simulink model "gm_soc_dvbs2_fpga"  (R2025b)
settings: Solver=VariableStepAuto  StartTime=0.0  StopTime=10.0  RelTol=1e-3
InitFcn:
  | soc_dvbs2_init;
undefined symbols (not defined in the file or in its folder): Add, coefficientsLog, coefficientsSqrt1, coefficientsSqrt2, dataBits, Deinterleaver, designMultirateFIR, noisePow, Shift, Short, soc_dvbs2_designFIRFilter, soc_dvbs2_txPacketBits, syncWord, txDataOut, txFiltCoeff, XData
libraries: simulink x304, hdlsllib x265, dspsigops x15, dsphdlfiltering2 x8, hdlmdlgenlib x6, dsphdlsigops2 x5, commseqgen3 x5, dsphdlmathfun2 x3, hwlogicconnlib x2, whdledac x2, commhdlcrc x2, whdlutilities x1
(part 36 of 36)

== system gm_soc_dvbs2_fpga/DVBS2/DVBS2 TxRx/DVB-S2 HDL Receiver/Synchronizer and PL Header Decoder/Time Frequency and Coarse Phase Synchronizer/Fine Frequency Synchronizer/Modified L and R Algorithm/L and R Algorithm 18 point/Compute R(m) for 13 to 18/Compute R(m)_3/Complex Multiplier ==
  In1 : Inport  OutDataTypeStr=fixdt(1, 16, 11)  PortDimensions=1  SampleTime=2.5e-07
      settings: SignalType=complex
  In2 : Inport  Port=2  OutDataTypeStr=fixdt(1, 16, 11)  PortDimensions=1  SampleTime=2.5e-07
      settings: SignalType=complex
  AddADn : Sum  Inputs=++|  OutDataTypeStr=fixdt(1, 33, 22)
  AddAUp : Sum  Inputs=|+-  OutDataTypeStr=fixdt(1, 33, 22)
  AddBCtr : Sum  Inputs=+|+  OutDataTypeStr=fixdt(1, 17, 11)
  AddBDn : Sum  Inputs=|+-  OutDataTypeStr=fixdt(1, 17, 11)
  AddBUp : Sum  Inputs=++|  OutDataTypeStr=fixdt(1, 17, 11)
  Complex to Real-Imag : ComplexToRealImag
  Complex to Real-Imag1 : ComplexToRealImag
  Delay{1..5,8..20} (18 alike) : Delay  DelayLength=1
  Delay{6..7,21..27} (9 alike) : Delay
  Product : Product  OutDataTypeStr=fixdt(1, 33, 22)
  Product1 : Product  OutDataTypeStr=fixdt(1, 33, 22)
  Product2 : Product  OutDataTypeStr=fixdt(1, 33, 22)
  Real-Imag to Complex : RealImagToComplex
  Out1 : Outport  SampleTime=2.5e-07  VectorParamsAs1DForOutWhenUnconnected=off
  wires:
  Delay9/1 -> AddBUp/1
  Delay26/1 -> Delay17/1
  [RE2] -> Delay14/1
  Delay5/1 -> Delay24/1
  [IM2] -> Delay10/1
  Delay24/1 -> Product2/2
  [RE2] -> Delay9/1
  Delay11/1 -> AddBCtr/1, Delay1/1
  In1/1 -> Complex to Real-Imag/1
  Delay10/1 -> AddBUp/2
  Delay12/1 -> Delay3/1
  In2/1 -> Complex to Real-Imag1/1
  Real-Imag to Complex/1 -> Out1/1
  Product2/1 -> Delay27/1
  AddBDn/1 -> Delay5/1
  [IM2] -> Delay15/1
  Complex to Real-Imag/1 -> Delay11/1
  AddAUp/1 -> Delay19/1
  Product/1 -> Delay25/1
  Complex to Real-Imag/2 -> Delay13/1
  Complex to Real-Imag1/1 -> [RE2]
  Product1/1 -> Delay26/1
  AddBCtr/1 -> Delay2/1
  Complex to Real-Imag1/2 -> [IM2]
  Delay14/1 -> AddBDn/1
  Delay15/1 -> AddBDn/2
  AddADn/1 -> Delay20/1
  AddBUp/1 -> Delay8/1
  Delay20/1 -> Real-Imag to Complex/2
  [IM2] -> Delay12/1
  Delay13/1 -> AddBCtr/2, Delay4/1
  Delay8/1 -> Delay6/1
  Delay1/1 -> Delay7/1
  Delay4/1 -> Delay23/1
  Delay6/1 -> Product/1
  Delay7/1 -> Product/2
  Delay2/1 -> Delay21/1
  Delay3/1 -> Delay22/1
  Delay23/1 -> Product2/1
  Delay21/1 -> Product1/1
  Delay22/1 -> Product1/2
  Delay25/1 -> Delay16/1
  Delay27/1 -> Delay18/1
  Delay16/1 -> AddAUp/1
  Delay17/1 -> AddAUp/2, AddADn/1
  Delay18/1 -> AddADn/2
  Delay19/1 -> Real-Imag to Complex/1

== system gm_soc_dvbs2_fpga/DVBS2/DVBS2 TxRx/DVB-S2 HDL Receiver/Synchronizer and PL Header Decoder/Time Frequency and Coarse Phase Synchronizer/Fine Frequency Synchronizer/Modified L and R Algorithm/L and R Algorithm 18 point/Compute R(m) for 13 to 18/Compute R(m)_4/Complex Multiplier ==
  In1 : Inport  OutDataTypeStr=fixdt(1, 16, 11)  PortDimensions=1  SampleTime=2.5e-07
      settings: SignalType=complex
  In2 : Inport  Port=2  OutDataTypeStr=fixdt(1, 16, 11)  PortDimensions=1  SampleTime=2.5e-07
      settings: SignalType=complex
  AddADn : Sum  Inputs=++|  OutDataTypeStr=fixdt(1, 33, 22)
  AddAUp : Sum  Inputs=|+-  OutDataTypeStr=fixdt(1, 33, 22)
  AddBCtr : Sum  Inputs=+|+  OutDataTypeStr=fixdt(1, 17, 11)
  AddBDn : Sum  Inputs=|+-  OutDataTypeStr=fixdt(1, 17, 11)
  AddBUp : Sum  Inputs=++|  OutDataTypeStr=fixdt(1, 17, 11)
  Complex to Real-Imag : ComplexToRealImag
  Complex to Real-Imag1 : ComplexToRealImag
  Delay{1..5,8..20} (18 alike) : Delay  DelayLength=1
  Delay{6..7,21..27} (9 alike) : Delay
  Product : Product  OutDataTypeStr=fixdt(1, 33, 22)
  Product1 : Product  OutDataTypeStr=fixdt(1, 33, 22)
  Product2 : Product  OutDataTypeStr=fixdt(1, 33, 22)
  Real-Imag to Complex : RealImagToComplex
  Out1 : Outport  SampleTime=2.5e-07  VectorParamsAs1DForOutWhenUnconnected=off
  wires:
  Delay9/1 -> AddBUp/1
  Product2/1 -> Delay27/1
  Delay7/1 -> Product/2
  AddBDn/1 -> Delay5/1
  [IM2] -> Delay15/1
  [RE2] -> Delay14/1
  Delay5/1 -> Delay24/1
  [IM2] -> Delay10/1
  AddAUp/1 -> Delay19/1
  Product/1 -> Delay25/1
  [RE2] -> Delay9/1
  Delay19/1 -> Real-Imag to Complex/1
  Delay11/1 -> Delay1/1, AddBCtr/1
  In1/1 -> Complex to Real-Imag/1
  Delay18/1 -> AddADn/2
  Delay10/1 -> AddBUp/2
  Delay12/1 -> Delay3/1
  In2/1 -> Complex to Real-Imag1/1
  Complex to Real-Imag/1 -> Delay11/1
  Complex to Real-Imag/2 -> Delay13/1
  Complex to Real-Imag1/1 -> [RE2]
  Complex to Real-Imag1/2 -> [IM2]
  Delay14/1 -> AddBDn/1
  Delay15/1 -> AddBDn/2
  AddBUp/1 -> Delay8/1
  Product1/1 -> Delay26/1
  AddBCtr/1 -> Delay2/1
  [IM2] -> Delay12/1
  Delay13/1 -> AddBCtr/2, Delay4/1
  Delay8/1 -> Delay6/1
  Delay1/1 -> Delay7/1
  Delay4/1 -> Delay23/1
  Delay6/1 -> Product/1
  Delay2/1 -> Delay21/1
  AddADn/1 -> Delay20/1
  Delay3/1 -> Delay22/1
  Delay23/1 -> Product2/1
  Delay24/1 -> Product2/2
  Delay21/1 -> Product1/1
  Delay22/1 -> Product1/2
  Delay25/1 -> Delay16/1
  Delay27/1 -> Delay18/1
  Delay16/1 -> AddAUp/1
  Delay26/1 -> Delay17/1
  Delay17/1 -> AddAUp/2, AddADn/1
  Delay20/1 -> Real-Imag to Complex/2
  Real-Imag to Complex/1 -> Out1/1

== system gm_soc_dvbs2_fpga/DVBS2/DVBS2 TxRx/DVB-S2 HDL Receiver/Synchronizer and PL Header Decoder/Time Frequency and Coarse Phase Synchronizer/Fine Frequency Synchronizer/Modified L and R Algorithm/L and R Algorithm 18 point/Compute R(m) for 13 to 18/Compute R(m)_5/Complex Multiplier ==
  In1 : Inport  OutDataTypeStr=fixdt(1, 16, 11)  PortDimensions=1  SampleTime=2.5e-07
      settings: SignalType=complex
  In2 : Inport  Port=2  OutDataTypeStr=fixdt(1, 16, 11)  PortDimensions=1  SampleTime=2.5e-07
      settings: SignalType=complex
  AddADn : Sum  Inputs=++|  OutDataTypeStr=fixdt(1, 33, 22)
  AddAUp : Sum  Inputs=|+-  OutDataTypeStr=fixdt(1, 33, 22)
  AddBCtr : Sum  Inputs=+|+  OutDataTypeStr=fixdt(1, 17, 11)
  AddBDn : Sum  Inputs=|+-  OutDataTypeStr=fixdt(1, 17, 11)
  AddBUp : Sum  Inputs=++|  OutDataTypeStr=fixdt(1, 17, 11)
  Complex to Real-Imag : ComplexToRealImag
  Complex to Real-Imag1 : ComplexToRealImag
  Delay{1..5,8..20} (18 alike) : Delay  DelayLength=1
  Delay{6..7,21..27} (9 alike) : Delay
  Product : Product  OutDataTypeStr=fixdt(1, 33, 22)
  Product1 : Product  OutDataTypeStr=fixdt(1, 33, 22)
  Product2 : Product  OutDataTypeStr=fixdt(1, 33, 22)
  Real-Imag to Complex : RealImagToComplex
  Out1 : Outport  SampleTime=2.5e-07  VectorParamsAs1DForOutWhenUnconnected=off
  wires:
  Delay9/1 -> AddBUp/1
  Delay7/1 -> Product/2
  [IM2] -> Delay15/1
  Delay26/1 -> Delay17/1
  [RE2] -> Delay14/1
  Delay5/1 -> Delay24/1
  [IM2] -> Delay10/1
  Delay24/1 -> Product2/2
  [RE2] -> Delay9/1
  Delay11/1 -> Delay1/1, AddBCtr/1
  In1/1 -> Complex to Real-Imag/1
  Delay10/1 -> AddBUp/2
  Delay12/1 -> Delay3/1
  In2/1 -> Complex to Real-Imag1/1
  Complex to Real-Imag/1 -> Delay11/1
  AddAUp/1 -> Delay19/1
  Product/1 -> Delay25/1
  Complex to Real-Imag/2 -> Delay13/1
  Complex to Real-Imag1/1 -> [RE2]
  Product1/1 -> Delay26/1
  AddBCtr/1 -> Delay2/1
  Complex to Real-Imag1/2 -> [IM2]
  Delay14/1 -> AddBDn/1
  Delay15/1 -> AddBDn/2
  AddADn/1 -> Delay20/1
  AddBUp/1 -> Delay8/1
  Delay20/1 -> Real-Imag to Complex/2
  [IM2] -> Delay12/1
  Delay13/1 -> AddBCtr/2, Delay4/1
  Real-Imag to Complex/1 -> Out1/1
  Product2/1 -> Delay27/1
  AddBDn/1 -> Delay5/1
  Delay8/1 -> Delay6/1
  Delay1/1 -> Delay7/1
  Delay4/1 -> Delay23/1
  Delay6/1 -> Product/1
  Delay2/1 -> Delay21/1
  Delay3/1 -> Delay22/1
  Delay23/1 -> Product2/1
  Delay21/1 -> Product1/1
  Delay22/1 -> Product1/2
  Delay25/1 -> Delay16/1
  Delay27/1 -> Delay18/1
  Delay16/1 -> AddAUp/1
  Delay17/1 -> AddADn/1, AddAUp/2
  Delay18/1 -> AddADn/2
  Delay19/1 -> Real-Imag to Complex/1

== system gm_soc_dvbs2_fpga/DVBS2/DVBS2 TxRx/DVB-S2 HDL Receiver/Synchronizer and PL Header Decoder/Time Frequency and Coarse Phase Synchronizer/Fine Frequency Synchronizer/Modified L and R Algorithm/L and R Algorithm 18 point/Compute R(m) for 13 to 18/Compute R(m)_6/Complex Multiplier ==
  In1 : Inport  OutDataTypeStr=fixdt(1, 16, 11)  PortDimensions=1  SampleTime=2.5e-07
      settings: SignalType=complex
  In2 : Inport  Port=2  OutDataTypeStr=fixdt(1, 16, 11)  PortDimensions=1  SampleTime=2.5e-07
      settings: SignalType=complex
  AddADn : Sum  Inputs=++|  OutDataTypeStr=fixdt(1, 33, 22)
  AddAUp : Sum  Inputs=|+-  OutDataTypeStr=fixdt(1, 33, 22)
  AddBCtr : Sum  Inputs=+|+  OutDataTypeStr=fixdt(1, 17, 11)
  AddBDn : Sum  Inputs=|+-  OutDataTypeStr=fixdt(1, 17, 11)
  AddBUp : Sum  Inputs=++|  OutDataTypeStr=fixdt(1, 17, 11)
  Complex to Real-Imag : ComplexToRealImag
  Complex to Real-Imag1 : ComplexToRealImag
  Delay{1..5,8..20} (18 alike) : Delay  DelayLength=1
  Delay{6..7,21..27} (9 alike) : Delay
  Product : Product  OutDataTypeStr=fixdt(1, 33, 22)
  Product1 : Product  OutDataTypeStr=fixdt(1, 33, 22)
  Product2 : Product  OutDataTypeStr=fixdt(1, 33, 22)
  Real-Imag to Complex : RealImagToComplex
  Out1 : Outport  SampleTime=2.5e-07  VectorParamsAs1DForOutWhenUnconnected=off
  wires:
  Delay9/1 -> AddBUp/1
  Product2/1 -> Delay27/1
  Delay7/1 -> Product/2
  AddBDn/1 -> Delay5/1
  [IM2] -> Delay15/1
  [RE2] -> Delay14/1
  [IM2] -> Delay10/1
  AddAUp/1 -> Delay19/1
  Product/1 -> Delay25/1
  Complex to Real-Imag/2 -> Delay13/1
  [RE2] -> Delay9/1
  In1/1 -> Complex to Real-Imag/1
  In2/1 -> Complex to Real-Imag1/1
  Delay18/1 -> AddADn/2
  Delay10/1 -> AddBUp/2
  Complex to Real-Imag/1 -> Delay11/1
  Complex to Real-Imag1/1 -> [RE2]
  Complex to Real-Imag1/2 -> [IM2]
  Delay14/1 -> AddBDn/1
  Delay15/1 -> AddBDn/2
  AddADn/1 -> Delay20/1
  AddBUp/1 -> Delay8/1
  Delay19/1 -> Real-Imag to Complex/1
  Delay11/1 -> AddBCtr/1, Delay1/1
  Product1/1 -> Delay26/1
  AddBCtr/1 -> Delay2/1
  [IM2] -> Delay12/1
  Delay13/1 -> AddBCtr/2, Delay4/1
  Delay8/1 -> Delay6/1
  Delay1/1 -> Delay7/1
  Delay12/1 -> Delay3/1
  Delay4/1 -> Delay23/1
  Delay5/1 -> Delay24/1
  Delay6/1 -> Product/1
  Delay2/1 -> Delay21/1
  Delay3/1 -> Delay22/1
  Delay23/1 -> Product2/1
  Delay24/1 -> Product2/2
  Delay21/1 -> Product1/1
  Delay22/1 -> Product1/2
  Delay25/1 -> Delay16/1
  Delay27/1 -> Delay18/1
  Delay26/1 -> Delay17/1
  Delay16/1 -> AddAUp/1
  Delay17/1 -> AddADn/1, AddAUp/2
  Delay20/1 -> Real-Imag to Complex/2
  Real-Imag to Complex/1 -> Out1/1

== system gm_soc_dvbs2_fpga/DVBS2/DVBS2 TxRx/DVB-S2 HDL Receiver/Synchronizer and PL Header Decoder/Time Frequency and Coarse Phase Synchronizer/Fine Frequency Synchronizer/Modified L and R Algorithm/L and R Algorithm 18 point/Compute R(m) for 7 to 12/Compute R(m)_1/Complex Multiplier ==
  In1 : Inport  OutDataTypeStr=fixdt(1, 16, 11)  PortDimensions=1  SampleTime=2.5e-07
      settings: SignalType=complex
  In2 : Inport  Port=2  OutDataTypeStr=fixdt(1, 16, 11)  PortDimensions=1  SampleTime=2.5e-07
      settings: SignalType=complex
  AddADn : Sum  Inputs=++|  OutDataTypeStr=fixdt(1, 33, 22)
  AddAUp : Sum  Inputs=|+-  OutDataTypeStr=fixdt(1, 33, 22)
  AddBCtr : Sum  Inputs=+|+  OutDataTypeStr=fixdt(1, 17, 11)
  AddBDn : Sum  Inputs=|+-  OutDataTypeStr=fixdt(1, 17, 11)
  AddBUp : Sum  Inputs=++|  OutDataTypeStr=fixdt(1, 17, 11)
  Complex to Real-Imag : ComplexToRealImag
  Complex to Real-Imag1 : ComplexToRealImag
  Delay{1..5,8..20} (18 alike) : Delay  DelayLength=1
  Delay{6..7,21..27} (9 alike) : Delay
  Product : Product  OutDataTypeStr=fixdt(1, 33, 22)
  Product1 : Product  OutDataTypeStr=fixdt(1, 33, 22)
  Product2 : Product  OutDataTypeStr=fixdt(1, 33, 22)
  Real-Imag to Complex : RealImagToComplex
  Out1 : Outport  SampleTime=2.5e-07  VectorParamsAs1DForOutWhenUnconnected=off
  wires:
  Delay9/1 -> AddBUp/1
  Delay7/1 -> Product/2
  [IM2] -> Delay15/1
  Delay26/1 -> Delay17/1
  [RE2] -> Delay14/1
  Delay5/1 -> Delay24/1
  [IM2] -> Delay10/1
  Product/1 -> Delay25/1
  Delay24/1 -> Product2/2
  [RE2] -> Delay9/1
  In1/1 -> Complex to Real-Imag/1
  In2/1 -> Complex to Real-Imag1/1
  Delay10/1 -> AddBUp/2
  Complex to Real-Imag/1 -> Delay11/1
  AddAUp/1 -> Delay19/1
  Complex to Real-Imag/2 -> Delay13/1
  Complex to Real-Imag1/1 -> [RE2]
  AddBCtr/1 -> Delay2/1
  Complex to Real-Imag1/2 -> [IM2]
  Delay14/1 -> AddBDn/1
  Delay15/1 -> AddBDn/2
  AddADn/1 -> Delay20/1
  AddBUp/1 -> Delay8/1
  Delay11/1 -> Delay1/1, AddBCtr/1
  Product1/1 -> Delay26/1
  [IM2] -> Delay12/1
  Delay13/1 -> AddBCtr/2, Delay4/1
  Real-Imag to Complex/1 -> Out1/1
  Product2/1 -> Delay27/1
  AddBDn/1 -> Delay5/1
  Delay8/1 -> Delay6/1
  Delay1/1 -> Delay7/1
  Delay12/1 -> Delay3/1
  Delay4/1 -> Delay23/1
  Delay6/1 -> Product/1
  Delay2/1 -> Delay21/1
  Delay3/1 -> Delay22/1
  Delay23/1 -> Product2/1
  Delay21/1 -> Product1/1
  Delay22/1 -> Product1/2
  Delay25/1 -> Delay16/1
  Delay27/1 -> Delay18/1
  Delay16/1 -> AddAUp/1
  Delay17/1 -> AddADn/1, AddAUp/2
  Delay18/1 -> AddADn/2
  Delay19/1 -> Real-Imag to Complex/1
  Delay20/1 -> Real-Imag to Complex/2

== system gm_soc_dvbs2_fpga/DVBS2/DVBS2 TxRx/DVB-S2 HDL Receiver/Synchronizer and PL Header Decoder/Time Frequency and Coarse Phase Synchronizer/Fine Frequency Synchronizer/Modified L and R Algorithm/L and R Algorithm 18 point/Compute R(m) for 7 to 12/Compute R(m)_2/Complex Multiplier ==
  In1 : Inport  OutDataTypeStr=fixdt(1, 16, 11)  PortDimensions=1  SampleTime=2.5e-07
      settings: SignalType=complex
  In2 : Inport  Port=2  OutDataTypeStr=fixdt(1, 16, 11)  PortDimensions=1  SampleTime=2.5e-07
      settings: SignalType=complex
  AddADn : Sum  Inputs=++|  OutDataTypeStr=fixdt(1, 33, 22)
  AddAUp : Sum  Inputs=|+-  OutDataTypeStr=fixdt(1, 33, 22)
  AddBCtr : Sum  Inputs=+|+  OutDataTypeStr=fixdt(1, 17, 11)
  AddBDn : Sum  Inputs=|+-  OutDataTypeStr=fixdt(1, 17, 11)
  AddBUp : Sum  Inputs=++|  OutDataTypeStr=fixdt(1, 17, 11)
  Complex to Real-Imag : ComplexToRealImag
  Complex to Real-Imag1 : ComplexToRealImag
  Delay{1..5,8..20} (18 alike) : Delay  DelayLength=1
  Delay{6..7,21..27} (9 alike) : Delay
  Product : Product  OutDataTypeStr=fixdt(1, 33, 22)
  Product1 : Product  OutDataTypeStr=fixdt(1, 33, 22)
  Product2 : Product  OutDataTypeStr=fixdt(1, 33, 22)
  Real-Imag to Complex : RealImagToComplex
  Out1 : Outport  SampleTime=2.5e-07  VectorParamsAs1DForOutWhenUnconnected=off
  wires:
  Delay9/1 -> AddBUp/1
  Real-Imag to Complex/1 -> Out1/1
  Product2/1 -> Delay27/1
  AddBDn/1 -> Delay5/1
  [IM2] -> Delay15/1
  [RE2] -> Delay14/1
  [IM2] -> Delay10/1
  AddAUp/1 -> Delay19/1
  Product/1 -> Delay25/1
  Complex to Real-Imag/2 -> Delay13/1
  [RE2] -> Delay9/1
  In1/1 -> Complex to Real-Imag/1
  In2/1 -> Complex to Real-Imag1/1
  Delay18/1 -> AddADn/2
  Delay10/1 -> AddBUp/2
  Complex to Real-Imag/1 -> Delay11/1
  Complex to Real-Imag1/1 -> [RE2]
  Product1/1 -> Delay26/1
  AddBCtr/1 -> Delay2/1
  [IM2] -> Delay12/1
  Complex to Real-Imag1/2 -> [IM2]
  Delay14/1 -> AddBDn/1
  Delay15/1 -> AddBDn/2
  AddADn/1 -> Delay20/1
  AddBUp/1 -> Delay8/1
  Delay19/1 -> Real-Imag to Complex/1
  Delay11/1 -> AddBCtr/1, Delay1/1
  Delay13/1 -> AddBCtr/2, Delay4/1
  Delay8/1 -> Delay6/1
  Delay1/1 -> Delay7/1
  Delay12/1 -> Delay3/1
  Delay4/1 -> Delay23/1
  Delay5/1 -> Delay24/1
  Delay6/1 -> Product/1
  Delay7/1 -> Product/2
  Delay2/1 -> Delay21/1
  Delay3/1 -> Delay22/1
  Delay23/1 -> Product2/1
  Delay24/1 -> Product2/2
  Delay21/1 -> Product1/1
  Delay22/1 -> Product1/2
  Delay25/1 -> Delay16/1
  Delay27/1 -> Delay18/1
  Delay16/1 -> AddAUp/1
  Delay26/1 -> Delay17/1
  Delay17/1 -> AddADn/1, AddAUp/2
  Delay20/1 -> Real-Imag to Complex/2

== system gm_soc_dvbs2_fpga/DVBS2/DVBS2 TxRx/DVB-S2 HDL Receiver/Synchronizer and PL Header Decoder/Time Frequency and Coarse Phase Synchronizer/Fine Frequency Synchronizer/Modified L and R Algorithm/L and R Algorithm 18 point/Compute R(m) for 7 to 12/Compute R(m)_3/Complex Multiplier ==
  In1 : Inport  OutDataTypeStr=fixdt(1, 16, 11)  PortDimensions=1  SampleTime=2.5e-07
      settings: SignalType=complex
  In2 : Inport  Port=2  OutDataTypeStr=fixdt(1, 16, 11)  PortDimensions=1  SampleTime=2.5e-07
      settings: SignalType=complex
  AddADn : Sum  Inputs=++|  OutDataTypeStr=fixdt(1, 33, 22)
  AddAUp : Sum  Inputs=|+-  OutDataTypeStr=fixdt(1, 33, 22)
  AddBCtr : Sum  Inputs=+|+  OutDataTypeStr=fixdt(1, 17, 11)
  AddBDn : Sum  Inputs=|+-  OutDataTypeStr=fixdt(1, 17, 11)
  AddBUp : Sum  Inputs=++|  OutDataTypeStr=fixdt(1, 17, 11)
  Complex to Real-Imag : ComplexToRealImag
  Complex to Real-Imag1 : ComplexToRealImag
  Delay{1..5,8..20} (18 alike) : Delay  DelayLength=1
  Delay{6..7,21..27} (9 alike) : Delay
  Product : Product  OutDataTypeStr=fixdt(1, 33, 22)
  Product1 : Product  OutDataTypeStr=fixdt(1, 33, 22)
  Product2 : Product  OutDataTypeStr=fixdt(1, 33, 22)
  Real-Imag to Complex : RealImagToComplex
  Out1 : Outport  SampleTime=2.5e-07  VectorParamsAs1DForOutWhenUnconnected=off
  wires:
  Delay9/1 -> AddBUp/1
  Product2/1 -> Delay27/1
  Delay7/1 -> Product/2
  [IM2] -> Delay15/1
  Delay26/1 -> Delay17/1
  [RE2] -> Delay14/1
  Delay5/1 -> Delay24/1
  [IM2] -> Delay10/1
  Product/1 -> Delay25/1
  Delay24/1 -> Product2/2
  [RE2] -> Delay9/1
  Delay19/1 -> Real-Imag to Complex/1
  Delay11/1 -> AddBCtr/1, Delay1/1
  In1/1 -> Complex to Real-Imag/1
  Delay18/1 -> AddADn/2
  Delay10/1 -> AddBUp/2
  Delay12/1 -> Delay3/1
  In2/1 -> Complex to Real-Imag1/1
  Complex to Real-Imag/1 -> Delay11/1
  AddAUp/1 -> Delay19/1
  Complex to Real-Imag/2 -> Delay13/1
  Complex to Real-Imag1/1 -> [RE2]
  AddBCtr/1 -> Delay2/1
  Complex to Real-Imag1/2 -> [IM2]
  Delay14/1 -> AddBDn/1
  Delay15/1 -> AddBDn/2
  AddBUp/1 -> Delay8/1
  Product1/1 -> Delay26/1
  [IM2] -> Delay12/1
  Delay13/1 -> AddBCtr/2, Delay4/1
  Real-Imag to Complex/1 -> Out1/1
  AddBDn/1 -> Delay5/1
  Delay8/1 -> Delay6/1
  Delay1/1 -> Delay7/1
  Delay4/1 -> Delay23/1
  Delay6/1 -> Product/1
  Delay2/1 -> Delay21/1
  AddADn/1 -> Delay20/1
  Delay3/1 -> Delay22/1
  Delay23/1 -> Product2/1
  Delay21/1 -> Product1/1
  Delay22/1 -> Product1/2
  Delay25/1 -> Delay16/1
  Delay27/1 -> Delay18/1
  Delay16/1 -> AddAUp/1
  Delay17/1 -> AddADn/1, AddAUp/2
  Delay20/1 -> Real-Imag to Complex/2

== system gm_soc_dvbs2_fpga/DVBS2/DVBS2 TxRx/DVB-S2 HDL Receiver/Synchronizer and PL Header Decoder/Time Frequency and Coarse Phase Synchronizer/Fine Frequency Synchronizer/Modified L and R Algorithm/L and R Algorithm 18 point/Compute R(m) for 7 to 12/Compute R(m)_4/Complex Multiplier ==
  In1 : Inport  OutDataTypeStr=fixdt(1, 16, 11)  PortDimensions=1  SampleTime=2.5e-07
      settings: SignalType=complex
  In2 : Inport  Port=2  OutDataTypeStr=fixdt(1, 16, 11)  PortDimensions=1  SampleTime=2.5e-07
      settings: SignalType=complex
  AddADn : Sum  Inputs=++|  OutDataTypeStr=fixdt(1, 33, 22)
  AddAUp : Sum  Inputs=|+-  OutDataTypeStr=fixdt(1, 33, 22)
  AddBCtr : Sum  Inputs=+|+  OutDataTypeStr=fixdt(1, 17, 11)
  AddBDn : Sum  Inputs=|+-  OutDataTypeStr=fixdt(1, 17, 11)
  AddBUp : Sum  Inputs=++|  OutDataTypeStr=fixdt(1, 17, 11)
  Complex to Real-Imag : ComplexToRealImag
  Complex to Real-Imag1 : ComplexToRealImag
  Delay{1..5,8..20} (18 alike) : Delay  DelayLength=1
  Delay{6..7,21..27} (9 alike) : Delay
  Product : Product  OutDataTypeStr=fixdt(1, 33, 22)
  Product1 : Product  OutDataTypeStr=fixdt(1, 33, 22)
  Product2 : Product  OutDataTypeStr=fixdt(1, 33, 22)
  Real-Imag to Complex : RealImagToComplex
  Out1 : Outport  SampleTime=2.5e-07  VectorParamsAs1DForOutWhenUnconnected=off
  wires:
  Delay9/1 -> AddBUp/1
  Delay24/1 -> Product2/2
  [RE2] -> Delay9/1
  Real-Imag to Complex/1 -> Out1/1
  Product2/1 -> Delay27/1
  AddBDn/1 -> Delay5/1
  [IM2] -> Delay15/1
  [RE2] -> Delay14/1
  [IM2] -> Delay10/1
  Delay11/1 -> AddBCtr/1, Delay1/1
  In1/1 -> Complex to Real-Imag/1
  Delay10/1 -> AddBUp/2
  In2/1 -> Complex to Real-Imag1/1
  Complex to Real-Imag/1 -> Delay11/1
  AddAUp/1 -> Delay19/1
  Product/1 -> Delay25/1
  Complex to Real-Imag/2 -> Delay13/1
  Complex to Real-Imag1/1 -> [RE2]
  Product1/1 -> Delay26/1
  AddBCtr/1 -> Delay2/1
  [IM2] -> Delay12/1
  Complex to Real-Imag1/2 -> [IM2]
  Delay14/1 -> AddBDn/1
  Delay15/1 -> AddBDn/2
  AddADn/1 -> Delay20/1
  AddBUp/1 -> Delay8/1
  Delay13/1 -> AddBCtr/2, Delay4/1
  Delay8/1 -> Delay6/1
  Delay1/1 -> Delay7/1
  Delay12/1 -> Delay3/1
  Delay4/1 -> Delay23/1
  Delay5/1 -> Delay24/1
  Delay6/1 -> Product/1
  Delay7/1 -> Product/2
  Delay2/1 -> Delay21/1
  Delay3/1 -> Delay22/1
  Delay23/1 -> Product2/1
  Delay21/1 -> Product1/1
  Delay22/1 -> Product1/2
  Delay25/1 -> Delay16/1
  Delay27/1 -> Delay18/1
  Delay16/1 -> AddAUp/1
  Delay26/1 -> Delay17/1
  Delay17/1 -> AddAUp/2, AddADn/1
  Delay18/1 -> AddADn/2
  Delay19/1 -> Real-Imag to Complex/1
  Delay20/1 -> Real-Imag to Complex/2

== system gm_soc_dvbs2_fpga/DVBS2/DVBS2 TxRx/DVB-S2 HDL Receiver/Synchronizer and PL Header Decoder/Time Frequency and Coarse Phase Synchronizer/Fine Frequency Synchronizer/Modified L and R Algorithm/L and R Algorithm 18 point/Compute R(m) for 7 to 12/Compute R(m)_5/Complex Multiplier ==
  In1 : Inport  OutDataTypeStr=fixdt(1, 16, 11)  PortDimensions=1  SampleTime=2.5e-07
      settings: SignalType=complex
  In2 : Inport  Port=2  OutDataTypeStr=fixdt(1, 16, 11)  PortDimensions=1  SampleTime=2.5e-07
      settings: SignalType=complex
  AddADn : Sum  Inputs=++|  OutDataTypeStr=fixdt(1, 33, 22)
  AddAUp : Sum  Inputs=|+-  OutDataTypeStr=fixdt(1, 33, 22)
  AddBCtr : Sum  Inputs=+|+  OutDataTypeStr=fixdt(1, 17, 11)
  AddBDn : Sum  Inputs=|+-  OutDataTypeStr=fixdt(1, 17, 11)
  AddBUp : Sum  Inputs=++|  OutDataTypeStr=fixdt(1, 17, 11)
  Complex to Real-Imag : ComplexToRealImag
  Complex to Real-Imag1 : ComplexToRealImag
  Delay{1..5,8..20} (18 alike) : Delay  DelayLength=1
  Delay{6..7,21..27} (9 alike) : Delay
  Product : Product  OutDataTypeStr=fixdt(1, 33, 22)
  Product1 : Product  OutDataTypeStr=fixdt(1, 33, 22)
  Product2 : Product  OutDataTypeStr=fixdt(1, 33, 22)
  Real-Imag to Complex : RealImagToComplex
  Out1 : Outport  SampleTime=2.5e-07  VectorParamsAs1DForOutWhenUnconnected=off
  wires:
  Delay9/1 -> AddBUp/1
  Product2/1 -> Delay27/1
  Delay7/1 -> Product/2
  [IM2] -> Delay15/1
  Delay26/1 -> Delay17/1
  [RE2] -> Delay14/1
  Delay5/1 -> Delay24/1
  [IM2] -> Delay10/1
  AddAUp/1 -> Delay19/1
  Product/1 -> Delay25/1
  [RE2] -> Delay9/1
  Delay19/1 -> Real-Imag to Complex/1
  Delay11/1 -> AddBCtr/1, Delay1/1
  In1/1 -> Complex to Real-Imag/1
  Delay18/1 -> AddADn/2
  Delay10/1 -> AddBUp/2
  Delay12/1 -> Delay3/1
  In2/1 -> Complex to Real-Imag1/1
  Complex to Real-Imag/1 -> Delay11/1
  Complex to Real-Imag/2 -> Delay13/1
  Complex to Real-Imag1/1 -> [RE2]
  Complex to Real-Imag1/2 -> [IM2]
  Delay14/1 -> AddBDn/1
  Delay15/1 -> AddBDn/2
  AddBUp/1 -> Delay8/1
  Product1/1 -> Delay26/1
  AddBCtr/1 -> Delay2/1
  [IM2] -> Delay12/1
  Delay13/1 -> AddBCtr/2, Delay4/1
  Real-Imag to Complex/1 -> Out1/1
  AddBDn/1 -> Delay5/1
  Delay8/1 -> Delay6/1
  Delay1/1 -> Delay7/1
  Delay4/1 -> Delay23/1
  Delay6/1 -> Product/1
  Delay2/1 -> Delay21/1
  AddADn/1 -> Delay20/1
  Delay3/1 -> Delay22/1
  Delay23/1 -> Product2/1
  Delay24/1 -> Product2/2
  Delay21/1 -> Product1/1
  Delay22/1 -> Product1/2
  Delay25/1 -> Delay16/1
  Delay27/1 -> Delay18/1
  Delay16/1 -> AddAUp/1
  Delay17/1 -> AddAUp/2, AddADn/1
  Delay20/1 -> Real-Imag to Complex/2

== system gm_soc_dvbs2_fpga/DVBS2/DVBS2 TxRx/DVB-S2 HDL Receiver/Synchronizer and PL Header Decoder/Time Frequency and Coarse Phase Synchronizer/Fine Frequency Synchronizer/Modified L and R Algorithm/L and R Algorithm 18 point/Compute R(m) for 7 to 12/Compute R(m)_6/Complex Multiplier ==
  In1 : Inport  OutDataTypeStr=fixdt(1, 16, 11)  PortDimensions=1  SampleTime=2.5e-07
      settings: SignalType=complex
  In2 : Inport  Port=2  OutDataTypeStr=fixdt(1, 16, 11)  PortDimensions=1  SampleTime=2.5e-07
      settings: SignalType=complex
  AddADn : Sum  Inputs=++|  OutDataTypeStr=fixdt(1, 33, 22)
  AddAUp : Sum  Inputs=|+-  OutDataTypeStr=fixdt(1, 33, 22)
  AddBCtr : Sum  Inputs=+|+  OutDataTypeStr=fixdt(1, 17, 11)
  AddBDn : Sum  Inputs=|+-  OutDataTypeStr=fixdt(1, 17, 11)
  AddBUp : Sum  Inputs=++|  OutDataTypeStr=fixdt(1, 17, 11)
  Complex to Real-Imag : ComplexToRealImag
  Complex to Real-Imag1 : ComplexToRealImag
  Delay{1..5,8..20} (18 alike) : Delay  DelayLength=1
  Delay{6..7,21..27} (9 alike) : Delay
  Product : Product  OutDataTypeStr=fixdt(1, 33, 22)
  Product1 : Product  OutDataTypeStr=fixdt(1, 33, 22)
  Product2 : Product  OutDataTypeStr=fixdt(1, 33, 22)
  Real-Imag to Complex : RealImagToComplex
  Out1 : Outport  SampleTime=2.5e-07  VectorParamsAs1DForOutWhenUnconnected=off
  wires:
  Delay9/1 -> AddBUp/1
  Delay7/1 -> Product/2
  [IM2] -> Delay15/1
  Delay26/1 -> Delay17/1
  [RE2] -> Delay14/1
  Delay5/1 -> Delay24/1
  [IM2] -> Delay10/1
  Delay18/1 -> AddADn/2
  Delay24/1 -> Product2/2
  [RE2] -> Delay9/1
  Delay11/1 -> AddBCtr/1, Delay1/1
  In1/1 -> Complex to Real-Imag/1
  Delay10/1 -> AddBUp/2
  Delay12/1 -> Delay3/1
  In2/1 -> Complex to Real-Imag1/1
  Complex to Real-Imag/1 -> Delay11/1
  AddAUp/1 -> Delay19/1
  Product/1 -> Delay25/1
  Complex to Real-Imag/2 -> Delay13/1
  Complex to Real-Imag1/1 -> [RE2]
  Product1/1 -> Delay26/1
  AddBCtr/1 -> Delay2/1
  Complex to Real-Imag1/2 -> [IM2]
  Delay14/1 -> AddBDn/1
  Delay15/1 -> AddBDn/2
  AddADn/1 -> Delay20/1
  AddBUp/1 -> Delay8/1
  Delay20/1 -> Real-Imag to Complex/2
  [IM2] -> Delay12/1
  Delay13/1 -> Delay4/1, AddBCtr/2
  Real-Imag to Complex/1 -> Out1/1
  Product2/1 -> Delay27/1
  AddBDn/1 -> Delay5/1
  Delay8/1 -> Delay6/1
  Delay1/1 -> Delay7/1
  Delay4/1 -> Delay23/1
  Delay6/1 -> Product/1
  Delay2/1 -> Delay21/1
  Delay3/1 -> Delay22/1
  Delay23/1 -> Product2/1
  Delay21/1 -> Product1/1
  Delay22/1 -> Product1/2
  Delay27/1 -> Delay18/1
  Delay25/1 -> Delay16/1
  Delay16/1 -> AddAUp/1
  Delay17/1 -> AddADn/1, AddAUp/2
  Delay19/1 -> Real-Imag to Complex/1

== matlab function gm_soc_dvbs2_fpga/DVBS2/DVBS2 TxRx/DVB-S2 HDL Receiver/Synchronizer and PL Header Decoder/Time Frequency and Coarse Phase Synchronizer/Time and Coarse Frequency Synchronizer/Symbol Synchronizer/Rate Handle/monostable/monostable ==
  data: trigger input; out output; nClocks parameter
function out = MonoStable(trigger,nClocks)
%#codegen

 persistent count;

 if isempty(count)
     count = fi(0,0,floor(log2(nClocks))+1,0,hdlfimath);
 end
 
 out = (count > 0);
 
 if (count > 0)
     count(:) = count - 1;
 end

 if trigger
     count(:) =  nClocks;
 end
 
end

== matlab function gm_soc_dvbs2_fpga/DVBS2/DVBS2 TxRx/DVB-S2 HDL Receiver/Demod Deinterleave and FECDecode/Discard Unsupported Frames/convertMODCOD/convertMODCOD ==
  data: modcod input; modIdx output; codIdx output
function [modIdx,codIdx] = convertMODCOD(modcod)
%#codegen

     modIdx = fi(0,0,2,0,hdlfimath);
     codIdx = fi(0,0,4,0,hdlfimath);
     if modcod < 12
         modIdx(:) = 0;
     elseif modcod < 18
         modIdx(:) = 1;
     elseif modcod < 24
         modIdx(:) = 2;
     else
         modIdx(:) = 3;
     end

     switch modcod
         case 1
             codIdx(:) = 0; % 1/4
         case 2
             codIdx(:) =  1; % 1/3
         case 3
             codIdx(:) =  2; % 2/5
         case 4
             codIdx(:) =  3; % 1/2
         case {5,12}
             codIdx(:) =  4; % 3/5
         case {6,13,18}
             codIdx(:) =  5; % 2/3
         case {7,14,19,24}
             codIdx(:) =  6; % 3/4
         case {8,20,25}
             codIdx(:) =  7; % 4/5
         case {9,15,21,26}
             codIdx(:) =  8; % 5/6
         case {10,16,22,27}
             codIdx(:) =  9; % 8/9
         case {11,17,23,28}
             codIdx(:) = 10; % 9/10
         otherwise
             codIdx(:) = 0; % use this as default

     end
end

== matlab function gm_soc_dvbs2_fpga/DVBS2/DVBS2 TxRx/DVB-S2 HDL Receiver/Stream Recovery/BB Decoder/Extract Data Field/Sample Discard Control/Sample Discard Control ==
  data: dataIn input; dataOut output; startIn input; endIn input; validIn input; startOut output; endOut output; validOut output
function [dataOut,startOut,endOut,validOut] = SampleDiscardControl(dataIn,startIn,endIn,validIn)
%#codegen

persistent active dataOutReg startOutReg endOutReg validOutReg;
     if isempty(active)
         active       = false;
         dataOutReg   = cast(0,'like',dataIn);
         startOutReg  = false;
         endOutReg    = false;
         validOutReg  = false;
     end
     
     dataOut    = dataOutReg;
     startOut   = startOutReg;
     endOut     = endOutReg;
     validOut   = validOutReg;

     if startIn
         active = true;
     end

     if active && validIn
         dataOutReg = dataIn;
         validOutReg = true;
     else
         dataOutReg(:)  = 0;
         validOutReg = false;
     end

     if endIn
         active = false;
     end

     startOutReg = startIn;
     endOutReg = endIn;
     

end

== matlab function gm_soc_dvbs2_fpga/DVBS2/DVBS2 TxRx/DVB-S2 HDL Receiver/Stream Recovery/BB Decoder/Extract Stream/Extract User Packet /Sample Discard Control/Sample Discard Control ==
  data: dataIn input; dataOut output; startIn input; endIn input; validIn input; startOut output; endOut output; validOut output
function [dataOut,startOut,endOut,validOut] = SampleDiscardControl(dataIn,startIn,endIn,validIn)
%#codegen

persistent active dataOutReg startOutReg endOutReg validOutReg;
     if isempty(active)
         active         = false;
         dataOutReg     = dataIn;
         dataOutReg(:)  = 0;
         startOutReg    = false;
         endOutReg      = false;
         validOutReg    = false;
     end
     
     dataOut    = dataOutReg;
     startOut   = startOutReg;
     endOut     = endOutReg;
     validOut   = validOutReg;

     if startIn
         active = true;
     end

     if active && validIn
         dataOutReg = dataIn;
         validOutReg = true;
     else
         dataOutReg(:)  = 0;
         validOutReg = false;
     end

     if endIn
         active = false;
     end

     startOutReg = startIn;
     endOutReg = endIn;
     

end

== matlab function gm_soc_dvbs2_fpga/DVBS2/DVBS2 TxRx/DVB-S2 HDL Receiver/Stream Recovery/BB Decoder/Extract Stream/Extract User Packet /Variable Count Limited HDL Counter/Variable Count Limited HDL Counter ==
  data: rst input; countToValue input; enb input; Hit output
function Hit = VariableCountLimitedHDLCounter(rst,countToValue,enb)
%#codegen

    persistent countState;
    if isempty(countState)
        countState = cast(0,'like',countToValue);
    end
    
%     count = countState;
    if enb
        Hit0 = (countState == 0);
        HitcountToValue = (countState == countToValue - 1);
        Hit = [Hit0;HitcountToValue];
    else
        Hit = false(2,1);
    end

    if rst
        countState(:) = 0;
    elseif enb
        if countState == countToValue - 1
            countState(:) = 0;
        else
            countState(:) = countState + 1;
        end
    end
end

== matlab function gm_soc_dvbs2_fpga/DVBS2/DVBS2 TxRx/DVB-S2 HDL Receiver/Demod Deinterleave and FECDecode/DVBS2 HDL Deinterleaver/Discard Out of  Frame samples/Discard Out of  Frame samples ==
  data: dataIn input; dataOut output; valid input; validOut output; reset input; fec input
function [dataOut,validOut] = fcn(dataIn,valid,reset,fec)
%#codegen
  
  COUNTMAX_NORMAL = 64800;
  COUNTMAX_SHORT = 16200;

  persistent count dataReg validReg;
  if isempty(count)
      count = fi(COUNTMAX_NORMAL,0,nextpow2(COUNTMAX_NORMAL),0,hdlfimath);
      validReg = false;
      dataReg = cast(0,'like',dataIn);
  end
  
  dataOut = dataReg;
  validOut = validReg;

  if fec
      COUNTMAX = fi(COUNTMAX_SHORT,0,nextpow2(COUNTMAX_NORMAL),0,hdlfimath);
  else
      COUNTMAX = fi(COUNTMAX_NORMAL,0,nextpow2(COUNTMAX_NORMAL),0,hdlfimath);
  end


  if valid && (count < COUNTMAX)
      count(:) = count + 1;
      dataReg = dataIn;
      validReg = valid;
  else
      dataReg(:) = 0;
      validReg = false;
  end
  
  if reset
      count(:) = 0;
  end


end

== matlab function gm_soc_dvbs2_fpga/DVBS2/DVBS2 TxRx/Channel/AWGN Generator/Unit Variance Gaussian Noise/SqrtImplementation/SqrtEval/RangeReduction/leadingZeroDetector ==
  data: x input; exp_f output
function exp_f=leadingZeroDetector(x)
%exp_e=31-length(dec2bin(x));
temp = 0;
flag=1.0e+09 *[

   0.000000002000000
   0.000000004000000
   0.000000008000000
   0.000000016000000
   0.000000032000000
   0.000000064000000
   0.000000128000000
   0.000000256000000
   0.000000512000000
   0.000001024000000
   0.000002048000000
   0.000004096000000
   0.000008192000000
   0.000016384000000
   0.000032768000000
   0.000065536000000
   0.000131072000000
   0.000262144000000
   0.000524288000000
   0.001048576000000
   0.002097152000000
   0.004194304000000
   0.008388608000000
   0.016777216000000
   0.033554432000000
   0.067108864000000
   0.134217728000000
   0.268435456000000
   0.536870912000000
   1.073741824000000
   2.147483648000000];

% else
%     while( )
%         temp = temp+1;
%         flag()=flag()*2;
%     end
% end
% 
% end
if(x == 0)
     temp = 31;
elseif (x*flag(1)>1)
        temp=1;
elseif (x*flag(2)>1)
        temp=2;
elseif (x*flag(3)>1)
        temp=3;
elseif (x*flag(4)>1)
        temp=4;
elseif (x*flag(5)>1)
        temp=5;
elseif (x*flag(6)>1)
        temp=6;
elseif (x*flag(7)>1)
        temp=7;
elseif (x*flag(8)>1)
        temp=8;
elseif (x*flag(9)>1)
        temp=9;
elseif (x*flag(10)>1)
        temp=10;
elseif (x*flag(11)>1)
        temp=11;
elseif (x*flag(12)>1)
        temp=12;
elseif (x*flag(13)>1)
        temp=13;
elseif (x*flag(14)>1)
        temp=14;
elseif (x*flag(15)>1)
        temp=15;
elseif (x*flag(16)>1)
        temp=16;
elseif (x*flag(17)>1)
        temp=17;
elseif (x*flag(18)>1)
        temp=18;
elseif (x*flag(19)>1)
        temp=19;
elseif (x*flag(20)>1)
        temp=20;
elseif (x*flag(21)>1)
        temp=21;
elseif (x*flag(22)>1)
        temp=22;
elseif (x*flag(23)>1)
        temp=23;
elseif (x*flag(24)>1)
        temp=24;
elseif (x*flag(25)>1)
        temp=25;
elseif (x*flag(26)>1)
        temp=26;
elseif (x*flag(27)>1)
        temp=27;
elseif (x*flag(28)>1)
        temp=28;
elseif (x*flag(29)>1)
        temp=29;
elseif (x*flag(30)>1)
        temp=30;              
end        
exp_f=uint8(temp);

== matlab function gm_soc_dvbs2_fpga/DVBS2/DVBS2 TxRx/DVB-S2 HDL Receiver/Demod Deinterleave and FECDecode/DVBS2 HDL Deinterleaver/RAM Address Generator/Read Offset Address/Read Offset Address Signals Generator/Read Offset Address Signals Generator ==
  data: maxR input; chkwrAddrEnd input; maxC input; modcodIs12 input; wrAddr input; curCorROut output; maxRorCOut output; curRorCOut output; modcodIs12Out output; startOut output; endOut output; wrEnb input; readValid output; isInterleave parameter
function [curCorROut,maxRorCOut,curRorCOut,modcodIs12Out,startOut,endOut,readValid] = readAddrCtrl(maxR,chkwrAddrEnd,maxC,modcodIs12,wrAddr,wrEnb,isInterleave)
%#codegen

    persistent rdEnb rdEnbOld startOutReg;
    persistent curR curC vMaxR vMaxC wrIdx rdIdx;
    persistent framCnt vModCodIs12;
    persistent curCorROutReg maxRorCOutReg curRorCOutReg modcodIs12OutReg;

    if isempty(rdEnb)
        rdEnb           = false;
%         rdEnbPrev       = false;
        rdEnbOld        = false;
        curR            = cast(0,'like',maxR);
        curC            = cast(0,'like',maxC);
        wrIdx           = fi(0,0,3,0,hdlfimath);
        rdIdx           = fi(0,0,3,0,hdlfimath);
        vMaxR           = cast(zeros(8,1),'like',maxR);
        vMaxC           = cast(zeros(8,1),'like',maxC);
        vModCodIs12     = false(8,1);
        startOutReg     = false;
        framCnt         = fi(0,0,3,0,hdlfimath);
        
        % XorY => Store X for Interleaver and Y for Deinterleaver
        if isInterleave        
            curCorROutReg   = curC;
            maxRorCOutReg   = vMaxR(1);
            curRorCOutReg   = curR;
        else
            curCorROutReg   = curR;
            maxRorCOutReg   = vMaxC(1);
            curRorCOutReg   = curC;
        end
        
        modcodIs12OutReg = vModCodIs12(1);
    end
    
    curCorROut   = curCorROutReg;
    maxRorCOut   = maxRorCOutReg;
    curRorCOut   = curRorCOutReg;
    modcodIs12Out = modcodIs12OutReg;
    readValid = rdEnbOld;
    startOut  = startOutReg; 
    
    endOut = false;
    if rdEnbOld
        if (isInterleave && (curC == (vMaxC(rdIdx+1)-1))) || (~isInterleave && (curR == (vMaxR(rdIdx+1)-1)))
            if isInterleave
                curC(:) = 0;
            else
                curR(:) = 0;
            end 
            if (~isInterleave && (curC == (vMaxC(rdIdx+1)-1))) || (isInterleave && (curR == (vMaxR(rdIdx+1)-1)))
                if ~isInterleave
                    curC(:) = 0;
                else
                    curR(:) = 0;
                end
                framCnt(:) = framCnt - 1;
                if framCnt == 0
                    rdEnb(:) = false;
                end
                endOut = true;
                if rdIdx == 7
                    rdIdx(:) = 0;
                else
                    rdIdx(:) = rdIdx + 1;
                end
            else
                if isInterleave
                    curR(:) = curR + 1;
                else
                    curC(:) = curC + 1;
                end
            end
        else
            if isInterleave
                curC(:) = curC + 1;
            else
                curR(:) = curR + 1;
            end
        end
    end
    
    if vModCodIs12(rdIdx+1) && curC == 0
        curCAdj = cast(2,'like',curC);
    elseif vModCodIs12(rdIdx+1) && curC == 2
        curCAdj = cast(0,'like',curC);
    else
        curCAdj = curC;
    end
    
    
    if isInterleave
        curCorROutReg    = curCAdj;
        maxRorCOutReg    = vMaxR(rdIdx+1);
        curRorCOutReg    = curR;
    else
        curCorROutReg    = curR;
        maxRorCOutReg    = vMaxC(rdIdx+1);
        curRorCOutReg    = curCAdj;
    end
    
    modcodIs12OutReg = vModCodIs12(rdIdx+1);

    startOutReg = rdEnb && (curR==0) && (curC==0);
    rdEnbOld = rdEnb;
%     rdEnbPrev = wrEnb && (wrAddr == chkwrAddrEnd);
    
    if wrEnb && (wrAddr == chkwrAddrEnd)
        framCnt(:) = framCnt + 1;
        rdEnb(:) = true;
        vModCodIs12(wrIdx+1) = modcodIs12;
        vMaxR(wrIdx+1) = maxR;
        vMaxC(wrIdx+1) = maxC;
        if wrIdx == 7
            wrIdx(:) = 0;
        else
            wrIdx(:) = wrIdx + 1;
        end
    end
    
end

== matlab function gm_soc_dvbs2_fpga/DVBS2/DVBS2 TxRx/Channel/AWGN Generator/Unit Variance Gaussian Noise/logImplementation/log/RangeReduction/leadingZeroDetector ==
  data: x input; exp_e output
function exp_e=leadingZeroDetector(x)
temp = 0;
flag=1.0e+14 *[0.000000000000020
   0.000000000000040
   0.000000000000080
   0.000000000000160
   0.000000000000320
   0.000000000000640
   0.000000000001280
   0.000000000002560
   0.000000000005120
   0.000000000010240
   0.000000000020480
   0.000000000040960
   0.000000000081920
   0.000000000163840
   0.000000000327680
   0.000000000655360
   0.000000001310720
   0.000000002621440
   0.000000005242880
   0.000000010485760
   0.000000020971520
   0.000000041943040
   0.000000083886080
   0.000000167772160
   0.000000335544320
   0.000000671088640
   0.000001342177280
   0.000002684354560
   0.000005368709120
   0.000010737418240
   0.000021474836480
   0.000042949672960
   0.000085899345920
   0.000171798691840
   0.000343597383680
   0.000687194767360
   0.001374389534720
   0.002748779069440
   0.005497558138880
   0.010995116277760
   0.021990232555520
   0.043980465111040
   0.087960930222080
   0.175921860444160
   0.351843720888320
   0.703687441776640
   1.407374883553280
   2.814749767106560];

% else
%     while( )
%         temp = temp+1;
%         flag()=flag()*2;
%     end
% end
% 
% end
if(x == 0)
     temp = 49;
elseif (x*flag(1)>1)
        temp=1;
elseif (x*flag(2)>1)
        temp=2;
elseif (x*flag(3)>1)
        temp=3;
elseif (x*flag(4)>1)
        temp=4;
elseif (x*flag(5)>1)
        temp=5;
elseif (x*flag(6)>1)
        temp=6;
elseif (x*flag(7)>1)
        temp=7;
elseif (x*flag(8)>1)
        temp=8;
elseif (x*flag(9)>1)
        temp=9;
elseif (x*flag(10)>1)
        temp=10;
elseif (x*flag(11)>1)
        temp=11;
elseif (x*flag(12)>1)
        temp=12;
elseif (x*flag(13)>1)
        temp=13;
elseif (x*flag(14)>1)
        temp=14;
elseif (x*flag(15)>1)
        temp=15;
elseif (x*flag(16)>1)
        temp=16;
elseif (x*flag(17)>1)
        temp=17;
elseif (x*flag(18)>1)
        temp=18;
elseif (x*flag(19)>1)
        temp=19;
elseif (x*flag(20)>1)
        temp=20;
elseif (x*flag(21)>1)
        temp=21;
elseif (x*flag(22)>1)
        temp=22;
elseif (x*flag(23)>1)
        temp=23;
elseif (x*flag(24)>1)
        temp=24;
elseif (x*flag(25)>1)
        temp=25;
elseif (x*flag(26)>1)
        temp=26;
elseif (x*flag(27)>1)
        temp=27;
elseif (x*flag(28)>1)
        temp=28;
elseif (x*flag(29)>1)
        temp=29;
elseif (x*flag(30)>1)
        temp=30;
elseif (x*flag(31)>1)
        temp=31;
elseif (x*flag(32)>1)
        temp=32;
elseif (x*flag(33)>1)
        temp=33;
elseif (x*flag(34)>1)
        temp=34;
elseif (x*flag(35)>1)
        temp=35;
elseif (x*flag(36)>1)
        temp=36;
elseif (x*flag(37)>1)
        temp=37;
elseif (x*flag(38)>1)
        temp=8;
elseif (x*flag(39)>1)
        temp=39;
elseif (x*flag(40)>1)
        temp=40;
elseif (x*flag(41)>1)
        temp=41;
elseif (x*flag(42)>1)
        temp=42;
elseif (x*flag(43)>1)
        temp=43;
elseif (x*flag(44)>1)
        temp=44;
elseif (x*flag(45)>1)
        temp=45;
elseif (x*flag(46)>1)
        temp=46;
elseif (x*flag(47)>1)
        temp=47; 
elseif (x*flag(48)>1)
        temp=48; 
end        
exp_e=uint8(temp);

== matlab function gm_soc_dvbs2_fpga/DVBS2/DVBS2 TxRx/DVB-S2 HDL Receiver/Synchronizer and PL Header Decoder/Source Encoding/MATLAB Function/MATLAB Function ==
  data: In input; out output; isdummy output
function [out,isdummy] = fcn(In)


if (In == 0)
    out = fi(0,0,2,0);
    isdummy = true;    
elseif (In <= 11)
    out = fi(0,0,2,0);
    isdummy = false;
elseif (In <= 17)
    out = fi(1,0,2,0);
    isdummy = false;
elseif (In <= 23)
    out = fi(2,0,2,0);
    isdummy = false;
elseif (In <= 28)
    out = fi(3,0,2,0);
    isdummy = false;
else
    out = fi(0,0,2,0);
    isdummy = true;
end

== matlab function gm_soc_dvbs2_fpga/DVBS2/DVBS2 TxRx/DVB-S2 HDL Receiver/Synchronizer and PL Header Decoder/Time Frequency and Coarse Phase Synchronizer/Time and Coarse Frequency Synchronizer/Frame Synchronizer/Pilot and Sync Pulse Indicator/ThresholdLimiter/ThresholdLimiter ==
  settings: fimath=hdlfimath
  data: x input; y output
function y = applyLowerLimit(x)
    % Apply a lower limit to the threshold.
    %#codegen
    
    % Threshold is computed by summing across 63 samples.
    % Set lower limit to be equivalent of all 63 samples
    % having their LSB set to 1 and all others set to 0. 
    lowerLimit = cast(64 * 2^-x.FractionLength, 'like', x); % use 64 for HDL
    
    if x < lowerLimit
        y = lowerLimit;
    else
        y = x;
    end
end

== matlab function gm_soc_dvbs2_fpga/DVBS2/DVBS2 TxRx/DVB-S2 HDL Receiver/Synchronizer and PL Header Decoder/Time Frequency and Coarse Phase Synchronizer/Time and Coarse Frequency Synchronizer/Symbol Synchronizer/Interpolation Control/Interpolation Control ==
  data: mu output; Delta input; Underflow output
function [mu,Underflow] = Interpolation_ctrl(Delta)
% Implementation of modulo-1 counter for interpolation control listed in
% Figure 8.4.19 of "Digital Communications - A Discrete-Time Approach"
% by Michael Rice. See design details in Chapter 8.4.3 of the same book.
% 
% Input:
%   Delta - Loop filter output. If loop is in lock, delta would be small
% Output:
%   Underflow - Indicator of counter underflow. This is the strobe signal
%               for downstream processing
%   mu - Difference between actual sampling instant and the optimal instant,
%        between zero and one
%#codegen

% countReg - Counter value delayed by 1 sample
% muReg - The estimated timing error normalized by half QPSK symbols

   mask = fi(1-2^(-10),1,11,10);
   
   persistent countReg underflowReg muReg;
   if isempty(countReg)
       countReg  = fi(0,1,11,10);
       muReg = fi(0,1,11,10);
       underflowReg = false;
   end
   
   
   Underflow = underflowReg;
   mu = muReg;   
   
   
   counter = bitand(mask,countReg)-Delta-fi(0.25,1,11,10); % decrementing counter
   
   % if countReg is a nonnegative number,
   % then mod(countReg,1) equals the fractional part of countReg
   if counter < 0
       underflowReg = true;
       muReg = bitshift(bitand(mask,countReg),2);
       countReg = fi(counter+1,1,11,10);% create underflow to counter
   else
       underflowReg = false;
       countReg = fi(counter,1,11,10);
   end
   


end

== matlab function gm_soc_dvbs2_fpga/DVBS2/DVBS2 TxRx/DVB-S2 HDL Receiver/Synchronizer and PL Header Decoder/Time Frequency and Coarse Phase Synchronizer/Time and Coarse Frequency Synchronizer/Symbol Synchronizer/Rate Handle/FIFO/MATLAB Function/MATLAB Function ==
  data: wr input; full output; rd input; empty output
function [full,empty] = fcn(wr,rd)
%#codegen
     
    WL = nextpow2(1024-1);
    maxCountVal = fi(2^(WL+1) - 1,0,WL+1,0);
    persistent count;
    if isempty(count)
        count = fi(0,0,WL+1,0,hdlfimath);
    end

   

    if wr
        if count == maxCountVal
            count(:) = 0;
        else
            count(:) = count + 1;
        end
    end
    if rd
        if count == 0
            count(:) = maxCountVal;
        else
            count(:) = count - 1;
        end
    end


    empty = (count == 0);
    full = (count > 2^WL-1);
    % ncount = count;

end
